simulink model "QD2_DroneStack_PID_R2023a"  (R2023a)
settings: Solver=ode1  StartTime=0.0  StopTime=inf  FixedStep=1/1000  RelTol=1e-3  EnableMultiTasking=on
InitFcn:
  | Motor_Mapping_7_Inch
model workspace (MAT data in the model file):
  target_system = 1
undefined symbols (not defined in the file): _Commander, datetime, HIL, KT, lf, log_, log_QD2_, m, Motor_Matrix, n, qc_get_step_size, s, saved_data
libraries: quarc_library x112, simulink x27, simulink_extras x3
(part 3 of 5)

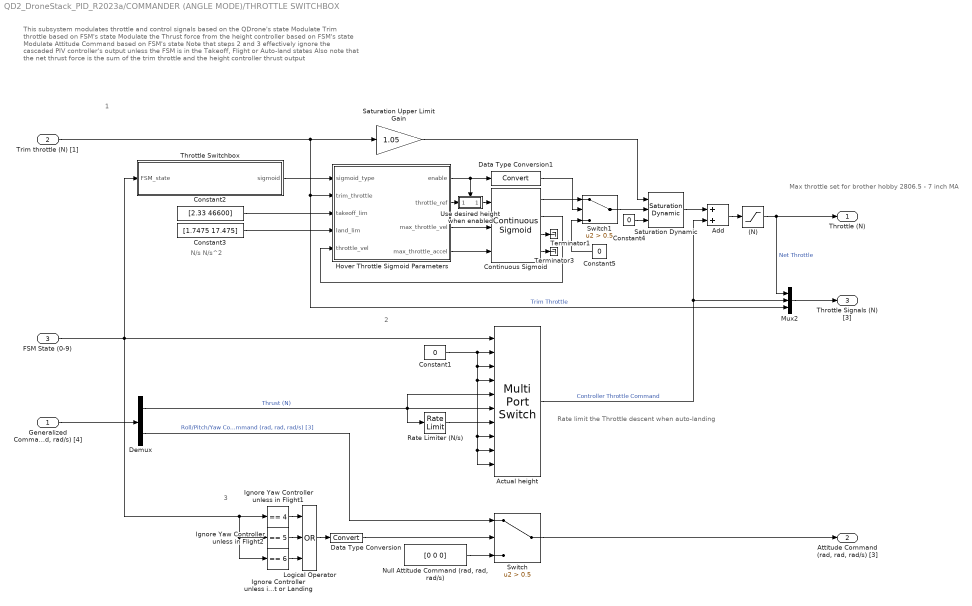
== system QD2_DroneStack_PID_R2023a/COMMANDER (ANGLE MODE)/THROTTLE SWITCHBOX  ==
  note: N/s N/s^2
  note: This subsystem modulates throttle and control signals based on the QDrone's state
      | Modulate Trim throttle based on FSM's state
      | Modulate the Thrust force from the height controller based on FSM's state
      | Modulate Attitude Command based on FSM's state
      |
      | Note that steps 2 and 3 effectively ignore the cascaded PIV controller's output unless the FSM is in the Takeoff, Flight or Auto-land states
      | Also note that the net thrust force is the sum of the trim throttle and the height controller thrust output
  note: Rate limit the Throttle descent when auto-landing
  note: 1
  note: 2
  note: 3
  note: Max throttle set for brother hobby 2806.5 - 7 inch MA
  "Generalized Command (N, rad, rad, rad/s) [4]" : Inport
  Trim throttle (N) [1] : Inport  Port=2
  FSM State (0-9) : Inport  Port=3
  (N) : Saturate  UpperLimit=58  LowerLimit=0
  Actual height : MultiPortSwitch  Inputs=9  SaturateOnIntegerOverflow=off  InputSameDT=off
  Add : Sum
  Constant1 : Constant  Value=0
  Constant2 : Constant  Value=[2.33 46600]
  Constant3 : Constant  Value=[1.7475 17.475]
  Constant4 : Constant  Value=0
  Constant5 : Constant  Value=0
  Continuous Sigmoid : quarc_library/Sources/Sigmoids/Continuous Sigmoid  params_source=External (input ports)  max_velocity=2  max_acceleration=10  initial_position=0  initial_velocity=0  hold_off=0.5  input_sample_time=-1  output_sample_time=qc_get_step_size
      settings: SourceProductName=QUARC Targets
  Data Type Conversion : DataTypeConversion  SaturateOnIntegerOverflow=off  RndMeth=Floor
  Data Type Conversion1 : DataTypeConversion  SaturateOnIntegerOverflow=off  RndMeth=Floor
  Demux : Demux  Outputs=[1 3]
  Hover Throttle Sigmoid Parameters : MATLAB Function  TreatAsAtomicUnit=on
  "Ignore Controller unless in Takeoff, Flight or Landing" : simulink/Logic and Bit Operations/Compare To Constant  relop===  const=6  OutDataTypeStr=boolean
  Ignore Yaw Controller unless in Flight1 : simulink/Logic and Bit Operations/Compare To Constant  relop===  const=4  OutDataTypeStr=boolean
  Ignore Yaw Controller unless in Flight2 : simulink/Logic and Bit Operations/Compare To Constant  relop===  const=5  OutDataTypeStr=boolean
  Logical Operator : Logic  Operator=OR  Inputs=3  AllPortsSameDT=off  OutDataTypeStr=boolean
  Mux2 : Mux  Inputs=3
  "Null Attitude Command (rad, rad, rad/s)" : Constant  Value=[0 0 0]
  Rate Limiter (N/s) : RateLimiter  RisingSlewLimit=100  FallingSlewLimit=-100  SampleTimeMode=inherited
  Saturation Dynamic : simulink/Discontinuities/Saturation Dynamic  OutMin=[]  OutMax=[]  OutDataTypeStr=Inherit: Same as second input  OutDataType=fixdt(1, 16)  OutScaling=2^-10  DoSatur=off
  Saturation Upper Limit Gain : Gain  Gain=1.05
  Switch : Switch  Criteria=u2 > Threshold  Threshold=0.5  SaturateOnIntegerOverflow=off  InputSameDT=off
  Switch1 : Switch  Criteria=u2 > Threshold  Threshold=0.5  SaturateOnIntegerOverflow=off  InputSameDT=off
  Terminator1 : Terminator
  Terminator3 : Terminator
  Throttle Switchbox : MATLAB Function  TreatAsAtomicUnit=on
  Use desired height when enabled : Subsystem  TreatAsAtomicUnit=on
  Throttle (N) : Outport  VectorParamsAs1DForOutWhenUnconnected=off
  "Attitude Command (rad, rad, rad/s) [3]" : Outport  Port=2  VectorParamsAs1DForOutWhenUnconnected=off
  Throttle Signals (N) [3] : Outport  Port=3  VectorParamsAs1DForOutWhenUnconnected=off
  wires:
  Rate Limiter (N/s)/1 -> Actual height/7
  Constant1/1 -> Actual height/2, Actual height/3, Actual height/4, Actual height/9, Actual height/10, Actual height/8
  Switch/1 -> "Attitude Command (rad, rad, rad/s) [3]"/1
  Constant5/1 -> Switch1/3
  Hover Throttle Sigmoid Parameters/2(throttle_ref) -> Use desired height when enabled/1(h_d (m) [1])
  Use desired height when enabled/1(Out1) -> Continuous Sigmoid/1
  Continuous Sigmoid/3 -> Terminator1/1
  Hover Throttle Sigmoid Parameters/1(enable) -> Use desired height when enabled/Enable, Data Type Conversion1/1
  Data Type Conversion1/1 -> Switch1/2
  Hover Throttle Sigmoid Parameters/3(max_throttle_vel) -> Continuous Sigmoid/2
  Continuous Sigmoid/4 -> Terminator3/1
  Continuous Sigmoid/1 -> Switch1/1
  Hover Throttle Sigmoid Parameters/4(max_throttle_accel) -> Continuous Sigmoid/3
  Constant2/1 -> Hover Throttle Sigmoid Parameters/3(takeoff_lim)
  Saturation Upper Limit Gain/1 -> Saturation Dynamic/1
  Throttle Switchbox/1(sigmoid) -> Hover Throttle Sigmoid Parameters/1(sigmoid_type)
  Trim throttle (N) [1]/1 -> Saturation Upper Limit Gain/1, Hover Throttle Sigmoid Parameters/2(trim_throttle), Mux2/3  "Trim Throttle"
  Switch1/1 -> Saturation Dynamic/2
  Constant3/1 -> Hover Throttle Sigmoid Parameters/4(land_lim)
  Saturation Dynamic/1 -> Add/1
  Constant4/1 -> Saturation Dynamic/3
  Continuous Sigmoid/2 -> Hover Throttle Sigmoid Parameters/5(throttle_vel)
  Demux/1 -> Actual height/5, Rate Limiter (N/s)/1, Actual height/6  "Thrust (N)"
  Logical Operator/1 -> Data Type Conversion/1
  "Ignore Controller unless in Takeoff, Flight or Landing"/1 -> Logical Operator/3
  FSM State (0-9)/1 -> Throttle Switchbox/1(FSM_state), Ignore Yaw Controller unless in Flight1/1, Ignore Yaw Controller unless in Flight2/1, "Ignore Controller unless in Takeoff, Flight or Landing"/1, Actual height/1
  Demux/2 -> Switch/1  "Roll/Pitch/Yaw Command (rad, rad, rad/s) [3]"
  Ignore Yaw Controller unless in Flight1/1 -> Logical Operator/1
  "Null Attitude Command (rad, rad, rad/s)"/1 -> Switch/3
  Data Type Conversion/1 -> Switch/2
  Ignore Yaw Controller unless in Flight2/1 -> Logical Operator/2
  Mux2/1 -> Throttle Signals (N) [3]/1
  "Generalized Command (N, rad, rad, rad/s) [4]"/1 -> Demux/1
  (N)/1 -> Throttle (N)/1, Mux2/1  "Net Throttle"
  Add/1 -> (N)/1
  Actual height/1 -> Add/2, Mux2/2  "Controller Throttle Command"

== system QD2_DroneStack_PID_R2023a/Communication/Detect Communication Loss ==
  note: Stream Loss: Check if the state is 2 and error is positive (error codes are negative). Otherwise issue a communication error.
      | OR
      | Data Loss: Check if the data is stale for a while (this is required because a connected stream may publish no new data). If stale, issue a communication error.
  State : Inport
  Error : Inport  Port=2
  Data Out : Inport  Port=3
  Clock1 : Clock
  Communication Loss : Scope  NumInputPorts=2
  Data Type Conversion4 : DataTypeConversion  SaturateOnIntegerOverflow=off  RndMeth=Floor
  Grab mission server time to detect flat lines : Selector  InputPortWidth=14  IndexOptions=Index vector (dialog)  Indices=[14]  OutputSizes=1
  Logical Operator4 : Logic  Operator=OR  AllPortsSameDT=off  OutDataTypeStr=boolean
  MATLAB Function : MATLAB Function  TreatAsAtomicUnit=on
  Terminator3 : Terminator
  Terminator5 : Terminator
  Threshold1 : quarc_library/Discontinuities/Threshold  operator=>=  param_src=Specify via dialog  threshold=0.5  duration=0.1
      settings: SourceProductName=QUARC Targets
  Threshold2 : quarc_library/Discontinuities/Threshold  operator=>=  param_src=Specify via dialog  threshold=0.5  duration=0.5
      settings: SourceProductName=QUARC Targets
  Communication Issue : Outport  VectorParamsAs1DForOutWhenUnconnected=off
  wires:
  Threshold2/1 -> Communication Loss/2, Logical Operator4/2
  Logical Operator4/1 -> Data Type Conversion4/1
  Threshold1/2 -> Terminator3/1
  MATLAB Function/2(data_loss) -> Threshold2/1
  MATLAB Function/1(stream_connection_loss) -> Threshold1/1
  Clock1/1 -> MATLAB Function/1(time)
  Threshold2/2 -> Terminator5/1
  Threshold1/1 -> Communication Loss/1, Logical Operator4/1
  Grab mission server time to detect flat lines/1 -> MATLAB Function/4(ms_time)
  Data Out/1 -> Grab mission server time to detect flat lines/1
  State/1 -> MATLAB Function/2(state)
  Error/1 -> MATLAB Function/3(error)
  Data Type Conversion4/1 -> Communication Issue/1

== system QD2_DroneStack_PID_R2023a/Communication/Triggered Subsystem ==
  Trigger : TriggerPort  VariantControl=(inherit)
  Constant : Constant
  commOK : Outport  InitialOutput=[0]
  wires:
  Constant/1 -> commOK/1

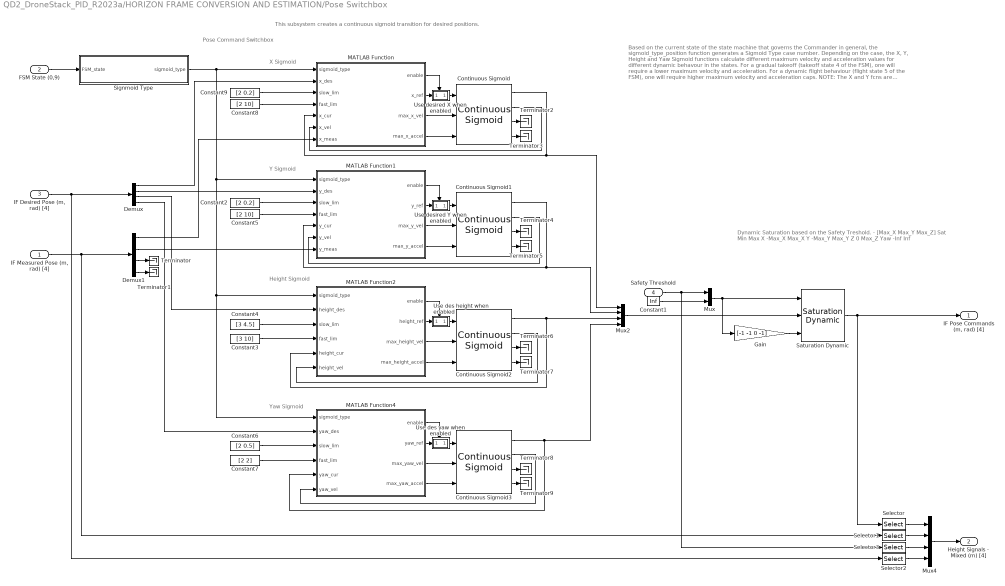
== system QD2_DroneStack_PID_R2023a/HORIZON FRAME CONVERSION AND ESTIMATION/Pose Switchbox ==
  note: Dynamic Saturation based on the Safety Treshold. - [Max_X Max_Y Max_Z]
      |
      | Sat Min Max
      | X -Max_X Max_X
      | Y -Max_Y Max_Y
      | Z 0 Max_Z
      | Yaw -Inf Inf
  note: Based on the current state of the state machine that governs the Commander in general,
      | the sigmoid_type_position function generates a Sigmoid Type case number. Depending on
      | the case, the X, Y, Height and Yaw Sigmoid functions calculate different maximum velocity
      | and acceleration values for different dynamic behavour in the states.
      |
      | For a gradual takeoff (takeoff state 4 of the FSM), one will require a lower maximum velocity
      | and acceleration. For a dynamic flight behaviour (flight state 5 of the FSM), one will require
      | higher maximum velocity and acceleration caps.
      |
      | NOTE: The X and Y fcns are logically identical due to the generally symmetric X and Y behaviour.
      | The Z and Yaw fcns are different.
  note: This subsystem creates a continuous sigmoid transition for desired positions.
  note: Height Sigmoid
  note: Pose Command Switchbox
  note: X Sigmoid
  note: Yaw Sigmoid
  note: Y Sigmoid
  "IF Measured Pose (m, rad) [4]" : Inport
  FSM State (0,9) : Inport  Port=2
  "IF Desired Pose (m, rad) [4]" : Inport  Port=3
  Safety Threshold : Inport  Port=4
  Constant1 : Constant  Value=Inf
  Constant2 : Constant  Value=[2 0.2]
  Constant3 : Constant  Value=[3 10]
  Constant4 : Constant  Value=[3 4.5]
  Constant5 : Constant  Value=[2 10]
  Constant6 : Constant  Value=[2 0.5]
  Constant7 : Constant  Value=[2 2]
  Constant8 : Constant  Value=[2 10]
  Constant9 : Constant  Value=[2 0.2]
  Continuous Sigmoid{,1..3} (4 alike) : quarc_library/Sources/Sigmoids/Continuous Sigmoid  params_source=External (input ports)  max_velocity=2  max_acceleration=10  initial_position=0  initial_velocity=0  hold_off=0.5  input_sample_time=-1  output_sample_time=qc_get_step_size
      settings: SourceProductName=QUARC Targets
  Demux : Demux
  Demux1 : Demux
  Gain : Gain  Gain=[-1 -1 0 -1]
  MATLAB Function : MATLAB Function  TreatAsAtomicUnit=on
  MATLAB Function1 : MATLAB Function  TreatAsAtomicUnit=on
  MATLAB Function2 : MATLAB Function  TreatAsAtomicUnit=on
  MATLAB Function4 : MATLAB Function  TreatAsAtomicUnit=on
  Mux : Mux  Inputs=2
  Mux2 : Mux
  Mux4 : Mux
  Saturation Dynamic : simulink/Discontinuities/Saturation Dynamic  OutMin=[]  OutMax=[]  OutDataTypeStr=Inherit: Same as second input  OutDataType=fixdt(1, 16)  OutScaling=2^-10  DoSatur=off
  Selector : Selector  InputPortWidth=4  IndexOptions=Index vector (dialog)  Indices=[3]  OutputSizes=1
  Selector1 : Selector  InputPortWidth=4  IndexOptions=Index vector (dialog)  Indices=[3]  OutputSizes=1
  Selector2 : Selector  InputPortWidth=4  IndexOptions=Index vector (dialog)  Indices=[3]  OutputSizes=1
  Selector3 : Selector  InputPortWidth=3  IndexOptions=Index vector (dialog)  Indices=[3]  OutputSizes=1
  Signmoid Type : MATLAB Function  TreatAsAtomicUnit=on
  Terminator{,1..9} (10 alike) : Terminator
  Use des height when enabled : Subsystem  TreatAsAtomicUnit=on
  Use des yaw when enabled : Subsystem  TreatAsAtomicUnit=on
  Use desired X when enabled : Subsystem  TreatAsAtomicUnit=on
  Use desired Y when enabled : Subsystem  TreatAsAtomicUnit=on
  "IF Pose Commands (m, rad) [4]" : Outport  VectorParamsAs1DForOutWhenUnconnected=off
  Height Signals - Mixed (m) [4] : Outport  Port=2  VectorParamsAs1DForOutWhenUnconnected=off
  wires:
  Constant4/1 -> MATLAB Function2/3(slow_lim)
  Constant3/1 -> MATLAB Function2/4(fast_lim)
  Selector/1 -> Mux4/1
  Selector1/1 -> Mux4/2
  Selector2/1 -> Mux4/4
  Selector3/1 -> Mux4/3
  Safety Threshold/1 -> Mux/1, Selector3/1
  Mux/1 -> Saturation Dynamic/1, Gain/1
  Constant1/1 -> Mux/2
  Saturation Dynamic/1 -> "IF Pose Commands (m, rad) [4]"/1, Selector/1
  Mux2/1 -> Saturation Dynamic/2
  Mux4/1 -> Height Signals - Mixed (m) [4]/1
  Gain/1 -> Saturation Dynamic/3
  Demux/2 -> MATLAB Function1/2(y_des)
  Use desired Y when enabled/1(Out1) -> Continuous Sigmoid1/1
  Use desired X when enabled/1(Out1) -> Continuous Sigmoid/1
  MATLAB Function2/3(max_height_vel) -> Continuous Sigmoid2/2
  Continuous Sigmoid3/3 -> Terminator8/1
  Demux1/4 -> Terminator1/1
  MATLAB Function4/1(enable) -> Use des yaw when enabled/Enable
  Use des yaw when enabled/1(Out1) -> Continuous Sigmoid3/1
  Continuous Sigmoid1/2 -> MATLAB Function1/6(y_vel)
  Constant2/1 -> MATLAB Function1/3(slow_lim)
  Constant6/1 -> MATLAB Function4/3(slow_lim)
  Demux1/1 -> MATLAB Function/7(x_meas)
  MATLAB Function1/2(y_ref) -> Use desired Y when enabled/1(h_d (m) [1])
  Demux/3 -> MATLAB Function2/2(height_des)
  Constant7/1 -> MATLAB Function4/4(fast_lim)
  Continuous Sigmoid1/4 -> Terminator5/1
  MATLAB Function1/1(enable) -> Use desired Y when enabled/Enable
  Continuous Sigmoid2/4 -> Terminator7/1
  Demux1/3 -> Terminator/1
  Signmoid Type/1(sigmoid_type) -> MATLAB Function/1(sigmoid_type), MATLAB Function1/1(sigmoid_type), MATLAB Function2/1(sigmoid_type), MATLAB Function4/1(sigmoid_type)
  MATLAB Function/3(max_x_vel) -> Continuous Sigmoid/2
  MATLAB Function2/1(enable) -> Use des height when enabled/Enable
  Constant9/1 -> MATLAB Function/3(slow_lim)
  Continuous Sigmoid2/2 -> MATLAB Function2/6(height_vel)
  Continuous Sigmoid1/1 -> MATLAB Function1/5(y_cur), Mux2/2
  MATLAB Function4/4(max_yaw_accel) -> Continuous Sigmoid3/3
  Demux/1 -> MATLAB Function/2(x_des)
  MATLAB Function1/3(max_y_vel) -> Continuous Sigmoid1/2
  Continuous Sigmoid3/2 -> MATLAB Function4/6(yaw_vel)
  MATLAB Function2/2(height_ref) -> Use des height when enabled/1(h_d (m) [1])
  MATLAB Function/4(max_x_accel) -> Continuous Sigmoid/3
  Use des height when enabled/1(Out1) -> Continuous Sigmoid2/1
  Continuous Sigmoid2/3 -> Terminator6/1
  Demux/4 -> MATLAB Function4/2(yaw_des)
  MATLAB Function1/4(max_y_accel) -> Continuous Sigmoid1/3
  MATLAB Function/1(enable) -> Use desired X when enabled/Enable
  Continuous Sigmoid3/4 -> Terminator9/1
  MATLAB Function4/2(yaw_ref) -> Use des yaw when enabled/1(h_d (m) [1])
  FSM State (0,9)/1 -> Signmoid Type/1(FSM_state)
  MATLAB Function2/4(max_height_accel) -> Continuous Sigmoid2/3
  Continuous Sigmoid/4 -> Terminator3/1
  Continuous Sigmoid/3 -> Terminator2/1
  Continuous Sigmoid/1 -> MATLAB Function/5(x_cur), Mux2/1
  Continuous Sigmoid/2 -> MATLAB Function/6(x_vel)
  MATLAB Function/2(x_ref) -> Use desired X when enabled/1(h_d (m) [1])
  Continuous Sigmoid3/1 -> MATLAB Function4/5(yaw_cur), Mux2/4
  MATLAB Function4/3(max_yaw_vel) -> Continuous Sigmoid3/2
  Continuous Sigmoid2/1 -> MATLAB Function2/5(height_cur), Mux2/3
  Demux1/2 -> MATLAB Function1/7(y_meas)
  Continuous Sigmoid1/3 -> Terminator4/1
  "IF Measured Pose (m, rad) [4]"/1 -> Demux1/1, Selector1/1
  "IF Desired Pose (m, rad) [4]"/1 -> Demux/1, Selector2/1
  Constant5/1 -> MATLAB Function1/4(fast_lim)
  Constant8/1 -> MATLAB Function/4(fast_lim)

== system QD2_DroneStack_PID_R2023a/QDrone 2 DAQ/Attitude Estimate from IMU Data ==
  IMU Data [12] : Inport
  For Each Subsystem - Iterate over IMU0 and IMU1 : Subsystem  TreatAsAtomicUnit=on
  Reshape into 2 columns for IMU0 and IMU1 : Reshape  OutputDimensionality=Customize  OutputDimensions=[6,2]
  Select Data for IMU0 : Selector  NumberOfDimensions=2  InputPortWidth=3  IndexOptions=Index vector (dialog),Index vector (dialog)  Indices=[1:9],[1]  OutputSizes=1,1
  Select Data for IMU1 : Selector  NumberOfDimensions=2  InputPortWidth=3  IndexOptions=Index vector (dialog),Index vector (dialog)  Indices=[1:9],[2]  OutputSizes=1,1
  "BF Estimated Attitude for IMU0 (rad, rad/s, rad/2^2) [9]" : Outport
  "BF Estimated Attitude for IMU1 (rad, rad/s, rad/2^2) [9]" : Outport  Port=2
  wires:
  Select Data for IMU1/1 -> "BF Estimated Attitude for IMU1 (rad, rad/s, rad/2^2) [9]"/1
  Select Data for IMU0/1 -> "BF Estimated Attitude for IMU0 (rad, rad/s, rad/2^2) [9]"/1
  For Each Subsystem - Iterate over IMU0 and IMU1/1("BF Estimated Attitude (rad, rad/s, rad/2^2) [9xn]") -> Select Data for IMU0/1, Select Data for IMU1/1
  Reshape into 2 columns for IMU0 and IMU1/1 -> For Each Subsystem - Iterate over IMU0 and IMU1/1(IMU Data [6xn])
  IMU Data [12]/1 -> Reshape into 2 columns for IMU0 and IMU1/1

== system QD2_DroneStack_PID_R2023a/QDrone 2 DAQ/Choose Motor Telemetry ==
  enable telemetry : Inport
  Bias1 : Bias  Bias=0:3  SaturateOnIntegerOverflow=off
  Constant1 : Constant  Value="[0 0 0 0; 1 0 0 0; 0 0 0 0; 0 1 0 0; 0 0 0 0; 0 0 1 0; 0 0 0 0;  0 0 0 1]"
  Constant2 : Constant  Value=8
  Gain : Gain  Gain=.7
  MATLAB Function : MATLAB Function  TreatAsAtomicUnit=on
  Selector : Selector  NumberOfDimensions=2  IndexMode=Zero-based  InputPortWidth=3  IndexOptions=Index vector (port),Select all  Indices=[1 3],1  OutputSizes=1,1
  Telemetry : Scope
  Zero-Order Hold1 : ZeroOrderHold  SampleTime=-1
  Motor telemetry select : Outport
  Motor telemetry index : Outport  Port=2
  wires:
  Constant2/1 -> MATLAB Function/2(n)
  Constant1/1 -> Selector/1
  Selector/1 -> Gain/1, Motor telemetry select/1
  enable telemetry/1 -> MATLAB Function/1(enable)
  Zero-Order Hold1/1 -> Motor telemetry index/1, Selector/2
  MATLAB Function/1(idx) -> Zero-Order Hold1/1
  Bias1/1 -> Telemetry/1
  Gain/1 -> Bias1/1

== system QD2_DroneStack_PID_R2023a/QDrone 2 DAQ/Construct ESC Speed ==
  ESC Data In [4] : Inport
  ESC Channel Select : Inport  Port=2
  For Each Subsystem - Construct ESC Signal : Subsystem  TreatAsAtomicUnit=on
  Memory : Memory  InitialCondition=zeros(1,4)
  ESC Data Out [4] : Outport
  wires:
  ESC Channel Select/1 -> For Each Subsystem - Construct ESC Signal/2(ESC Channel)
  ESC Data In [4]/1 -> For Each Subsystem - Construct ESC Signal/1(ESC Data In [4])
  Memory/1 -> For Each Subsystem - Construct ESC Signal/3(ESC Previous Data [4])
  For Each Subsystem - Construct ESC Signal/1(ESC Data Out [4]) -> Memory/1, ESC Data Out [4]/1

== system QD2_DroneStack_PID_R2023a/QDrone 2 DAQ/Construct ESC Temperature ==
  ESC Data In [4] : Inport
  ESC Channel Select : Inport  Port=2
  For Each Subsystem - Construct ESC Signal : Subsystem  TreatAsAtomicUnit=on
  Memory : Memory  InitialCondition=zeros(1,4)
  ESC Data Out [4] : Outport
  wires:
  ESC Channel Select/1 -> For Each Subsystem - Construct ESC Signal/2(ESC Channel)
  ESC Data In [4]/1 -> For Each Subsystem - Construct ESC Signal/1(ESC Data In [4])
  Memory/1 -> For Each Subsystem - Construct ESC Signal/3(ESC Previous Data [4])
  For Each Subsystem - Construct ESC Signal/1(ESC Data Out [4]) -> Memory/1, ESC Data Out [4]/1

== system QD2_DroneStack_PID_R2023a/QDrone 2 DAQ/Construct ESC Voltage ==
  ESC Data In [4] : Inport
  ESC Channel Select : Inport  Port=2
  For Each Subsystem - Construct ESC Signal : Subsystem  TreatAsAtomicUnit=on
  Memory : Memory  InitialCondition=zeros(1,4)
  ESC Data Out [4] : Outport
  wires:
  For Each Subsystem - Construct ESC Signal/1(ESC Data Out [4]) -> ESC Data Out [4]/1, Memory/1
  Memory/1 -> For Each Subsystem - Construct ESC Signal/3(ESC Previous Data [4])
  ESC Data In [4]/1 -> For Each Subsystem - Construct ESC Signal/1(ESC Data In [4])
  ESC Channel Select/1 -> For Each Subsystem - Construct ESC Signal/2(ESC Channel)

== system QD2_DroneStack_PID_R2023a/QDrone 2 DAQ/Detect ESC Problems ==
  ESC Telemetry Enabled : Inport
  ESC Channel Request [4] : Inport  Port=2
  ESC Channel Reported [4] : Inport  Port=3
  AND : Logic  IconShape=distinctive  AllPortsSameDT=off  OutDataTypeStr=boolean
  Compare To Constant : simulink/Logic and Bit Operations/Compare To Constant  relop=>=  const=20  OutDataTypeStr=boolean
  Constant : Constant  Value=200
  Delay{,1..3} (4 alike) : Delay
  Demux{,1..2,8} (4 alike) : Demux
  ESC Channel Mismatrch : Scope  NumInputPorts=4
  ESC Channel Mismatrch Count : Scope  NumInputPorts=4
  ESC Channel Selection Index : Scope  NumInputPorts=4
  For Each Subsystem : Subsystem  TreatAsAtomicUnit=on
  MATLAB Function : MATLAB Function  TreatAsAtomicUnit=on
  Mux : Mux
  Mux{1..4} (4 alike) : Mux  Inputs=2
  ESC Comm Problem [4] : Outport
  wires:
  Mux1/1 -> ESC Channel Selection Index/4
  Mux2/1 -> ESC Channel Selection Index/3
  Mux3/1 -> ESC Channel Selection Index/2
  Mux4/1 -> ESC Channel Selection Index/1
  Demux2/4 -> Mux4/2
  Demux2/3 -> Mux3/2
  Demux2/2 -> Mux2/2
  Demux2/1 -> Mux1/2
  ESC Telemetry Enabled/1 -> AND/2
  Compare To Constant/1 -> ESC Comm Problem [4]/1
  MATLAB Function/1(n) -> Demux1/1, Compare To Constant/1
  Demux1/2 -> ESC Channel Mismatrch Count/3
  Demux1/1 -> ESC Channel Mismatrch Count/4
  Demux1/3 -> ESC Channel Mismatrch Count/2
  Demux1/4 -> ESC Channel Mismatrch Count/1
  Constant/1 -> MATLAB Function/2(buffer_size)
  Demux8/4 -> ESC Channel Mismatrch/1
  Demux8/3 -> ESC Channel Mismatrch/2
  Demux8/1 -> ESC Channel Mismatrch/4
  Demux8/2 -> ESC Channel Mismatrch/3
  AND/1 -> Demux8/1, MATLAB Function/1(u)
  For Each Subsystem/1(mismatched [4]) -> AND/1
  Mux/1 -> For Each Subsystem/1(Channel Requested [4])
  Delay/1 -> Mux/4, Mux4/1
  Delay1/1 -> Mux/3, Mux3/1
  Delay3/1 -> Mux1/1, Mux/1
  Delay2/1 -> Mux/2, Mux2/1
  ESC Channel Request [4]/1 -> Demux/1
  Demux/4 -> Delay/1
  Demux/3 -> Delay1/1
  Demux/2 -> Delay2/1
  Demux/1 -> Delay3/1
  ESC Channel Reported [4]/1 -> For Each Subsystem/2(Channel Reported [4]), Demux2/1

== system QD2_DroneStack_PID_R2023a/QDrone 2 DAQ/Enabled Subsystem - Write ESC Commands ==
  DShot Raw [4] : Inport
  Enable : EnablePort
  HIL Write PWM : quarc_library/Data Acquisition/Generic/Immediate I//O/HIL Write PWM  object_name=HIL-1  channels=[0:3]  sample_time=-1  active=off  vector_input=on
      settings: AttributesFormatString=(%<object_name>)  SourceProductName=QUARC Targets
  wires:
  DShot Raw [4]/1 -> HIL Write PWM/1

== system QD2_DroneStack_PID_R2023a/QDrone 2 DAQ/Generate LED Pattern ==
  ESC States : Inport
  Blue Blue : Constant  Value=[0 0 1 0 0 1]
  Green Green : Constant  Value=[0 1 0 0 1 0]
  LED OFF : Constant  Value=[ 0 0 0 0 0 0]
  Multiport Switch : MultiPortSwitch  DataPortOrder=Specify indices  DataPortIndices={0,1,2,3,4,5,77,88,99}  DataPortForDefault=Additional data port  DiagnosticForDefault=Warning  SaturateOnIntegerOverflow=off  InputSameDT=off
  Red Blue : Constant  Value="[ 1 0 0 0 0 1   ]"
  Red Red : Constant  Value=[ 1 0 0 1 0 0]
  Red Yellow : Constant  Value="[ 1 0 0 1 1 0  ]"
  Yellow Blue : Constant  Value="[ 1 1 0 0 0 1  ]"
  Yellow Green : Constant  Value="[ 1 1 0 0 1 0  ]"
  Yellow Red : Constant  Value="[ 1 1 0 1 0 0  ]"
  Yellow Yellow : Constant  Value="[ 1 1 0 1 1 0  ]"
  LED Command : Outport
  wires:
  Red Yellow/1 -> Multiport Switch/6
  Yellow Red/1 -> Multiport Switch/5
  Yellow Green/1 -> Multiport Switch/3
  Green Green/1 -> Multiport Switch/7
  LED OFF/1 -> Multiport Switch/11
  Yellow Blue/1 -> Multiport Switch/8
  Red Blue/1 -> Multiport Switch/9
  Yellow Yellow/1 -> Multiport Switch/2
  Red Red/1 -> Multiport Switch/10
  Blue Blue/1 -> Multiport Switch/4
  ESC States/1 -> Multiport Switch/1
  Multiport Switch/1 -> LED Command/1

== system QD2_DroneStack_PID_R2023a/QDrone 2 DAQ/Monitor Battery Level ==
  note: Monitor Battery Level.
      | Flag Low Battery Error if
      | Battery level dips below
      | threshold for specified
      | threshold time period.
  Battery (V) : Inport
  AND : Logic  IconShape=distinctive  AllPortsSameDT=off  OutDataTypeStr=boolean
  Battery Low Time Threshold (s) : Constant  Value=0.3
  Constant : Constant  Value=0.5
  Data Type Conversion : DataTypeConversion  SaturateOnIntegerOverflow=off  RndMeth=Floor
  Data Type Conversion1 : DataTypeConversion  SaturateOnIntegerOverflow=off  RndMeth=Floor
  Greater than minimum expected voltage (Valid Battery Reading) : simulink/Logic and Bit Operations/Compare To Constant  relop=>  const=0.5  OutDataTypeStr=boolean
  Less than minimum threshold voltage (Battery level too low) : simulink/Logic and Bit Operations/Compare To Constant  relop=<=  const=14  OutDataTypeStr=boolean
  Terminator : Terminator
  Threshold : quarc_library/Discontinuities/Threshold  operator=>=  param_src=External input port  threshold=0  duration=0
      settings: SourceProductName=QUARC Targets
  Triggered Subsystem - Latching Flag : Subsystem  TreatAsAtomicUnit=on
  Low Battery : Outport
  wires:
  Data Type Conversion1/1 -> Low Battery/1
  Triggered Subsystem - Latching Flag/1(Out1) -> Data Type Conversion1/1
  Threshold/1 -> Triggered Subsystem - Latching Flag/Trigger
  Threshold/2 -> Terminator/1
  Data Type Conversion/1 -> Threshold/1
  Battery Low Time Threshold (s)/1 -> Threshold/3
  Constant/1 -> Threshold/2
  AND/1 -> Data Type Conversion/1
  Greater than minimum expected voltage (Valid Battery Reading)/1 -> AND/1
  Less than minimum threshold voltage (Battery level too low)/1 -> AND/2
  Battery (V)/1 -> Greater than minimum expected voltage (Valid Battery Reading)/1, Less than minimum threshold voltage (Battery level too low)/1

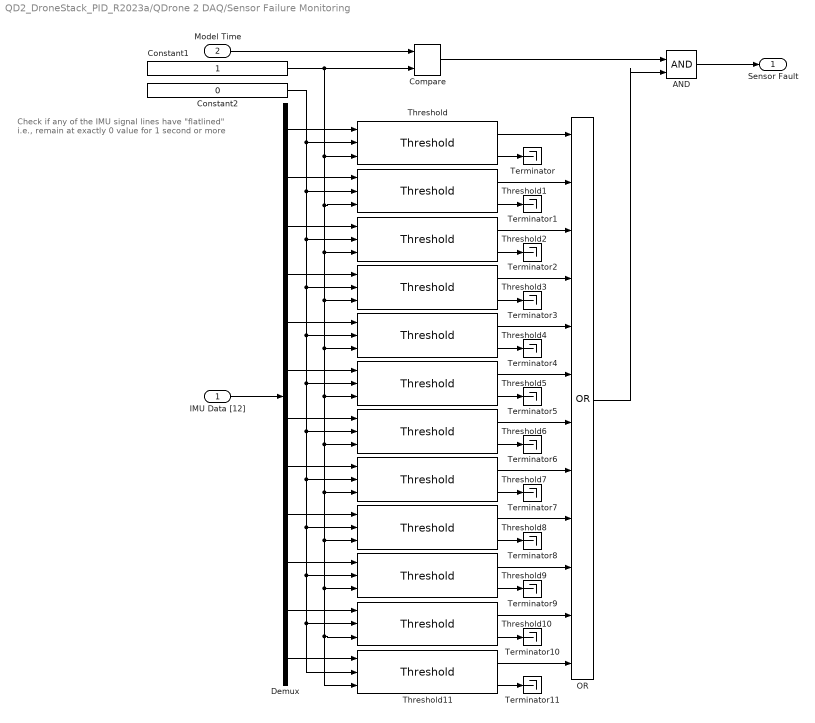
== system QD2_DroneStack_PID_R2023a/QDrone 2 DAQ/Sensor Failure Monitoring ==
  note: Check if any of the IMU signal lines have "flatlined"
      | i.e., remain at exactly 0 value for 1 second or more
  IMU Data [12] : Inport
  Model Time : Inport  Port=2
  AND : Logic  IconShape=distinctive  AllPortsSameDT=off  OutDataTypeStr=boolean
  Compare : quarc_library/Logic Operations/Compare  operator=>=  output_data_type=boolean
      settings: SourceProductName=QUARC Targets
  Constant1 : Constant
  Constant2 : Constant  Value=0
  Demux : Demux  Outputs=12
  OR : Logic  Operator=OR  Inputs=12  AllPortsSameDT=off  OutDataTypeStr=boolean
  Terminator{,1..11} (12 alike) : Terminator
  Threshold{,1..11} (12 alike) : quarc_library/Discontinuities/Threshold  operator===  param_src=External input port  threshold=0  duration=1
      settings: SourceProductName=QUARC Targets
  Sensor Fault : Outport
  wires:
  AND/1 -> Sensor Fault/1
  OR/1 -> AND/2
  Compare/1 -> AND/1
  Threshold11/2 -> Terminator11/1
  Threshold10/2 -> Terminator10/1
  Threshold9/2 -> Terminator9/1
  Threshold8/2 -> Terminator8/1
  Threshold7/2 -> Terminator7/1
  Threshold6/2 -> Terminator6/1
  Threshold5/2 -> Terminator5/1
  Threshold4/2 -> Terminator4/1
  Threshold3/2 -> Terminator3/1
  Threshold2/2 -> Terminator2/1
  Threshold1/2 -> Terminator1/1
  Threshold/2 -> Terminator/1
  Threshold11/1 -> OR/12
  Threshold10/1 -> OR/11
  Threshold9/1 -> OR/10
  Threshold8/1 -> OR/9
  Threshold7/1 -> OR/8
  Threshold6/1 -> OR/7
  Threshold5/1 -> OR/6
  Threshold4/1 -> OR/5
  Threshold3/1 -> OR/4
  Threshold2/1 -> OR/3
  Threshold1/1 -> OR/2
  Threshold/1 -> OR/1
  Demux/12 -> Threshold11/1
  Demux/11 -> Threshold10/1
  Demux/10 -> Threshold9/1
  Demux/9 -> Threshold8/1
  Demux/8 -> Threshold7/1
  Demux/7 -> Threshold6/1
  Demux/6 -> Threshold5/1
  Demux/5 -> Threshold4/1
  Demux/4 -> Threshold3/1
  Demux/3 -> Threshold2/1
  IMU Data [12]/1 -> Demux/1
  Constant2/1 -> Threshold/2, Threshold11/2, Threshold10/2, Threshold9/2, Threshold8/2, Threshold7/2, Threshold6/2, Threshold5/2, Threshold4/2, Threshold3/2, Threshold2/2, Threshold1/2
  Demux/2 -> Threshold1/1
  Demux/1 -> Threshold/1
  Constant1/1 -> Compare/2, Threshold/3, Threshold4/3, Threshold11/3, Threshold10/3, Threshold9/3, Threshold8/3, Threshold7/3, Threshold6/3, Threshold5/3, Threshold3/3, Threshold2/3, Threshold1/3
  Model Time/1 -> Compare/1

== system QD2_DroneStack_PID_R2023a/QDrone 2 DAQ/Timing Monitors ==
  note: ToF Range Rate (25 Hz)
  note: Optical Flow Rate (100 Hz)
  note: Base Model Rate (1kHz)
  Computation Time : quarc_library/Sources/Time/Computation Time  sample_time=qc_get_step_size  use_model=on  use_cpu_time=off
  Computation Time1 : quarc_library/Sources/Time/Computation Time  sample_time=0.01  use_model=on  use_cpu_time=off
  Computation Time2 : quarc_library/Sources/Time/Computation Time  sample_time=0.04  use_model=on  use_cpu_time=off
  Mux : Mux  Inputs=2
  Mux1 : Mux  Inputs=2
  Mux2 : Mux  Inputs=2
  Mux3 : Mux  Inputs=3
  Rate Transition{,1..3} (4 alike) : RateTransition
  Sample Time : quarc_library/Sources/Time/Sample Time  Priority=-99  sample_time=qc_get_step_size
  Sample Time1 : quarc_library/Sources/Time/Sample Time  Priority=-99  sample_time=0.01
  Sample Time2 : quarc_library/Sources/Time/Sample Time  Priority=-99  sample_time=0.04
  Timing Check : Scope  NumInputPorts=3
  Timings : Outport
  wires:
  Rate Transition3/1 -> Mux2/2
  Rate Transition2/1 -> Mux2/1
  Rate Transition1/1 -> Mux1/2
  Rate Transition/1 -> Mux1/1
  Mux3/1 -> Timings/1
  Mux2/1 -> Mux3/3, Timing Check/3
  Mux/1 -> Mux3/1, Timing Check/1
  Mux1/1 -> Timing Check/2, Mux3/2
  Sample Time2/1 -> Rate Transition3/1
  Computation Time2/1 -> Rate Transition2/1
  Computation Time1/1 -> Rate Transition/1
  Sample Time1/1 -> Rate Transition1/1
  Sample Time/1 -> Mux/2
  Computation Time/1 -> Mux/1

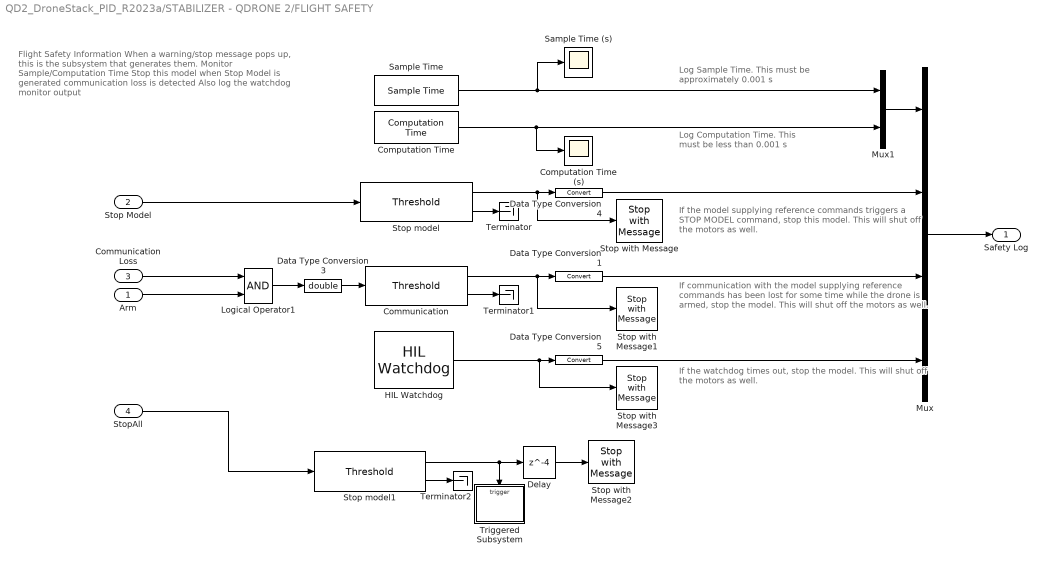
== system QD2_DroneStack_PID_R2023a/STABILIZER - QDRONE 2/FLIGHT SAFETY ==
  note: If the watchdog times out, stop the model. This will shut off the motors as well.
  note: If communication with the model supplying reference commands has been lost for some time while the drone is armed, stop the model. This will shut off the motors as well.
  note: If the model supplying reference commands triggers a STOP MODEL command, stop this model. This will shut off the motors as well.
  note: Log Computation Time. This must be less than 0.001 s
  note: Log Sample Time. This must be approximately 0.001 s
  note: Flight Safety Information
      |
      | When a warning/stop message pops up, this is the subsystem
      | that generates them.
      |
      | Monitor Sample/Computation Time
      | Stop this model
      | when Stop Model is generated
      | communication loss is detected
      | Also log the watchdog monitor output
  Arm : Inport
  Stop Model : Inport  Port=2
  Communication Loss : Inport  Port=3
  StopAll : Inport  Port=4
  Communication : quarc_library/Discontinuities/Threshold  operator=>=  param_src=Specify via dialog  threshold=0.5  duration=1
      settings: SourceProductName=QUARC Targets
  Computation Time : quarc_library/Sources/Time/Computation Time  sample_time=qc_get_step_size  use_model=on  use_cpu_time=off
  Computation Time (s) : Scope
  Data Type Conversion1 : DataTypeConversion  SaturateOnIntegerOverflow=off  RndMeth=Floor
  Data Type Conversion3 : DataTypeConversion  OutDataTypeStr=double  SaturateOnIntegerOverflow=off  RndMeth=Floor
  Data Type Conversion4 : DataTypeConversion  SaturateOnIntegerOverflow=off  RndMeth=Floor
  Data Type Conversion5 : DataTypeConversion  SaturateOnIntegerOverflow=off  RndMeth=Floor
  Delay : Delay  DelayLength=4
  HIL Watchdog : quarc_library/Data Acquisition/Generic/Watchdog/HIL Watchdog  object_name=HIL-1  timeout=0.1  sample_time=qc_get_step_size  active=off
      settings: AttributesFormatString=(%<object_name>)  SourceProductName=QUARC Targets
  Logical Operator1 : Logic  AllPortsSameDT=off  OutDataTypeStr=boolean
  Mux : Mux
  Mux1 : Mux  Inputs=2
  Sample Time : quarc_library/Sources/Time/Sample Time  Priority=-99  sample_time=qc_get_step_size
  Sample Time (s) : Scope
  Stop model : quarc_library/Discontinuities/Threshold  operator=>=  param_src=Specify via dialog  threshold=0.5  duration=0.2
      settings: SourceProductName=QUARC Targets
  Stop model1 : quarc_library/Discontinuities/Threshold  operator=>=  param_src=Specify via dialog  threshold=0.5  duration=1
      settings: SourceProductName=QUARC Targets
  Stop with Message : quarc_library/Sinks/Error Handling/Stop with Message  message_type=Fixed error message  message_icon=Information  message=QDrone Stabilizer: Commander Terminated
  Stop with Message1 : quarc_library/Sinks/Error Handling/Stop with Message  message_type=Fixed error message  message_icon=Warning  message=QDrone Stabilizer: Communication with Commander lost
  Stop with Message2 : quarc_library/Sinks/Error Handling/Stop with Message  message_type=Fixed error message  message_icon=Information  message=QDrone Stabilizer stopped from Mission Server
  Stop with Message3 : quarc_library/Sinks/Error Handling/Stop with Message  message_type=Fixed error message  message_icon=Information  message=QDrone Stabilizer: HIL Watchdog timer expired
  Terminator : Terminator
  Terminator1 : Terminator
  Terminator2 : Terminator
  Triggered Subsystem : Subsystem  TreatAsAtomicUnit=on
  Safety Log : Outport  VectorParamsAs1DForOutWhenUnconnected=off
  wires:
  Data Type Conversion5/1 -> Mux/4
  Mux1/1 -> Mux/1
  Communication Loss/1 -> Logical Operator1/1
  Data Type Conversion3/1 -> Communication/1
  Communication/1 -> Stop with Message1/1, Data Type Conversion1/1
  Arm/1 -> Logical Operator1/2
  Data Type Conversion1/1 -> Mux/3
  Logical Operator1/1 -> Data Type Conversion3/1
  Communication/2 -> Terminator1/1
  Stop Model/1 -> Stop model/1
  Stop model/1 -> Stop with Message/1, Data Type Conversion4/1
  Stop model/2 -> Terminator/1
  HIL Watchdog/1 -> Data Type Conversion5/1, Stop with Message3/1
  Data Type Conversion4/1 -> Mux/2
  Sample Time/1 -> Mux1/1, Sample Time (s)/1
  Computation Time/1 -> Mux1/2, Computation Time (s)/1
  Mux/1 -> Safety Log/1
  StopAll/1 -> Stop model1/1
  Stop model1/1 -> Delay/1, Triggered Subsystem/Trigger
  Stop model1/2 -> Terminator2/1
  Delay/1 -> Stop with Message2/1

== system QD2_DroneStack_PID_R2023a/COMMANDER (ANGLE MODE)/STATE MACHINE SIGNALS/Generate Extra Messages for Console ==
  time (s) : Inport
  Signal Triggers : Inport  Port=2
  Boolean Edge-Based Triggered Print : Subsystem  TreatAsAtomicUnit=on
  Matrix Concatenate : Concatenate  NumInputs=3  Mode=Multidimensional array  ConcatenateDimension=2
  String Constant12 : quarc_library/Strings/String Constant  string_value=DRONE DISARMED  evaluate_string=off  string_type=text  max_length=80  sample_time=inf  variable_size=off
      settings: AttributesFormatString="\"DRONE DISARMED\""  SourceProductName=QUARC Targets
  String Constant13 : quarc_library/Strings/String Constant  string_value=DRONE LANDING  evaluate_string=off  string_type=text  max_length=80  sample_time=inf  variable_size=off
      settings: AttributesFormatString="\"DRONE LANDING\""  SourceProductName=QUARC Targets
  String Constant16 : quarc_library/Strings/String Constant  string_value=INITIALIZATION FINISHED  evaluate_string=off  string_type=text  max_length=80  sample_time=inf  variable_size=off
      settings: AttributesFormatString="\"INITIALIZATION FINISHED\""  SourceProductName=QUARC Targets
  Terminator : Terminator
  wires:
  Matrix Concatenate/1 -> Boolean Edge-Based Triggered Print/2(Message)
  time (s)/1 -> Boolean Edge-Based Triggered Print/3(time (s))
  Signal Triggers/1 -> Boolean Edge-Based Triggered Print/1(Signal Enable)
  String Constant16/1 -> Matrix Concatenate/1
  String Constant12/1 -> Matrix Concatenate/2
  String Constant13/1 -> Matrix Concatenate/3
  Boolean Edge-Based Triggered Print/1(Out1) -> Terminator/1

== system QD2_DroneStack_PID_R2023a/COMMANDER (ANGLE MODE)/STATE MACHINE SIGNALS/Generate State Messages for Console ==
  time (s) : Inport
  DroneState [1-9] : Inport  Port=2
  Detect Change : simulink/Logic and Bit Operations/Detect Change  vinit=0  OutDataTypeStr=boolean
  Multiport Switch : MultiPortSwitch  Inputs=9  SaturateOnIntegerOverflow=off  InputSameDT=off
  String Constant1 : quarc_library/Strings/String Constant  string_value=DRONE ARMED  evaluate_string=off  string_type=text  max_length=80  sample_time=inf  variable_size=off
      settings: AttributesFormatString="\"DRONE ARMED\""  SourceProductName=QUARC Targets
  String Constant2 : quarc_library/Strings/String Constant  string_value=DRONE TAKEOFF THROTTLE  evaluate_string=off  string_type=text  max_length=80  sample_time=inf  variable_size=off
      settings: AttributesFormatString="\"DRONE TAKEOFF THROTTLE\""  SourceProductName=QUARC Targets
  String Constant3 : quarc_library/Strings/String Constant  string_value=DRONE TAKEOFF HEIGHT STATE  evaluate_string=off  string_type=text  max_length=80  sample_time=inf  variable_size=off
      settings: AttributesFormatString="\"DRONE TAKEOFF HEIGHT STATE\""  SourceProductName=QUARC Targets
  String Constant4 : quarc_library/Strings/String Constant  string_value=ERROR - DRONE EMERGENCY STOP  evaluate_string=off  string_type=text  max_length=80  sample_time=inf  variable_size=off
      settings: AttributesFormatString="\"ERROR - DRONE EMERGENCY STOP\""  SourceProductName=QUARC Targets
  String Constant5 : quarc_library/Strings/String Constant  string_value=DRONE IDLE - WAITING TO BE ARMED  evaluate_string=off  string_type=text  max_length=80  sample_time=inf  variable_size=off
      settings: AttributesFormatString="\"DRONE IDLE - WAITING TO BE ARMED\""  SourceProductName=QUARC Targets
  String Constant6 : quarc_library/Strings/String Constant  string_value=DRONE IS IN FLIGHT STATE  evaluate_string=off  string_type=text  max_length=80  sample_time=inf  variable_size=off
      settings: AttributesFormatString="\"DRONE IS IN FLIGHT STATE\""  SourceProductName=QUARC Targets
  String Constant7 : quarc_library/Strings/String Constant  string_value=EMERGENCY STOP WAS PRESSED ON JOYSTICK  evaluate_string=off  string_type=text  max_length=80  sample_time=inf  variable_size=off
      settings: AttributesFormatString="\"EMERGENCY STOP WAS PRESSED ON JOYSTICK\""  SourceProductName=QUARC Targets
  String Constant8 : quarc_library/Strings/String Constant  string_value=FLIGHT FINISHED DRONE IS DISABLED  evaluate_string=off  string_type=text  max_length=80  sample_time=inf  variable_size=off
      settings: AttributesFormatString="\"FLIGHT FINISHED DRONE IS DISABLED\""  SourceProductName=QUARC Targets
  String Constant9 : quarc_library/Strings/String Constant  string_value=DRONE IS AUTO LANDING  evaluate_string=off  string_type=text  max_length=80  sample_time=inf  variable_size=off
      settings: AttributesFormatString="\"DRONE IS AUTO LANDING\""  SourceProductName=QUARC Targets
  Triggered Subsystem : Subsystem  TreatAsAtomicUnit=on
  wires:
  DroneState [1-9]/1 -> Multiport Switch/1, Triggered Subsystem/1(Value), Detect Change/1
  Multiport Switch/1 -> Triggered Subsystem/3(Message)
  time (s)/1 -> Triggered Subsystem/2(Time (s))
  String Constant1/1 -> Multiport Switch/3
  String Constant2/1 -> Multiport Switch/4
  String Constant3/1 -> Multiport Switch/5
  String Constant6/1 -> Multiport Switch/6
  String Constant9/1 -> Multiport Switch/7
  String Constant4/1 -> Multiport Switch/8
  String Constant7/1 -> Multiport Switch/9
  String Constant8/1 -> Multiport Switch/10
  String Constant5/1 -> Multiport Switch/2
  Detect Change/1 -> Triggered Subsystem/Trigger

== system QD2_DroneStack_PID_R2023a/COMMANDER (ANGLE MODE)/STATE MACHINE SIGNALS/Generate Warning Messages for Console ==
  time (s) : Inport
  errors [8] : Inport  Port=2
  Boolean Value-Based Triggered Print : Subsystem  TreatAsAtomicUnit=on
  Matrix Concatenate : Concatenate  NumInputs=9  Mode=Multidimensional array  ConcatenateDimension=2
  String Constant : quarc_library/Strings/String Constant  string_value=Commander: Low Battery  evaluate_string=off  string_type=text  max_length=80  sample_time=inf  variable_size=off
      settings: AttributesFormatString="\"Commander: Low Battery\""  SourceProductName=QUARC Targets
  String Constant1 : quarc_library/Strings/String Constant  string_value=Commander: Sensor Failure  evaluate_string=off  string_type=text  max_length=80  sample_time=inf  variable_size=off
      settings: AttributesFormatString="\"Commander: Sensor Failure\""  SourceProductName=QUARC Targets
  String Constant2 : quarc_library/Strings/String Constant  string_value=Commander: Host Stream Issue / Problem with communication  evaluate_string=off  string_type=text  max_length=80  sample_time=inf  variable_size=off
      settings: AttributesFormatString="\"Commander: Host Stream Issue / Problem with communication\""  SourceProductName=QUARC Targets
  String Constant3 : quarc_library/Strings/String Constant  string_value=Commander: Joystick Issue  evaluate_string=off  string_type=text  max_length=80  sample_time=inf  variable_size=off
      settings: AttributesFormatString="\"Commander: Joystick Issue\""  SourceProductName=QUARC Targets
  String Constant4 : quarc_library/Strings/String Constant  string_value=Commander: Optitrack isn't tracking  evaluate_string=off  string_type=text  max_length=80  sample_time=inf  variable_size=off
      settings: AttributesFormatString="\"Commander: Optitrack isn't tracking\""  SourceProductName=QUARC Targets
  String Constant5 : quarc_library/Strings/String Constant  string_value=Commander: Flying low  evaluate_string=off  string_type=text  max_length=80  sample_time=inf  variable_size=off
      settings: AttributesFormatString="\"Commander: Flying low\""  SourceProductName=QUARC Targets
  String Constant6 : quarc_library/Strings/String Constant  string_value=Commander: Flying high  evaluate_string=off  string_type=text  max_length=80  sample_time=inf  variable_size=off
      settings: AttributesFormatString="\"Commander: Flying high\""  SourceProductName=QUARC Targets
  String Constant7 : quarc_library/Strings/String Constant  string_value=Commander: Emergency Stop Triggered  evaluate_string=off  string_type=text  max_length=80  sample_time=inf  variable_size=off
      settings: AttributesFormatString="\"Commander: Emergency Stop Triggered\""  SourceProductName=QUARC Targets
  String Constant8 : quarc_library/Strings/String Constant  string_value=Commander: Takeoff triggered before armed drone  evaluate_string=off  string_type=text  max_length=80  sample_time=inf  variable_size=off
      settings: AttributesFormatString="\"Commander: Takeoff triggered before armed drone\""  SourceProductName=QUARC Targets
  Terminator : Terminator
  wires:
  String Constant8/1 -> Matrix Concatenate/5
  String Constant4/1 -> Matrix Concatenate/6
  String Constant5/1 -> Matrix Concatenate/7
  String Constant6/1 -> Matrix Concatenate/8
  String Constant7/1 -> Matrix Concatenate/9
  Boolean Value-Based Triggered Print/1(Out1) -> Terminator/1
  String Constant3/1 -> Matrix Concatenate/4
  String Constant2/1 -> Matrix Concatenate/3
  String Constant1/1 -> Matrix Concatenate/2
  String Constant/1 -> Matrix Concatenate/1
  Matrix Concatenate/1 -> Boolean Value-Based Triggered Print/2(Message)
  errors [8]/1 -> Boolean Value-Based Triggered Print/1(Signal Enable)
  time (s)/1 -> Boolean Value-Based Triggered Print/3(time (s))

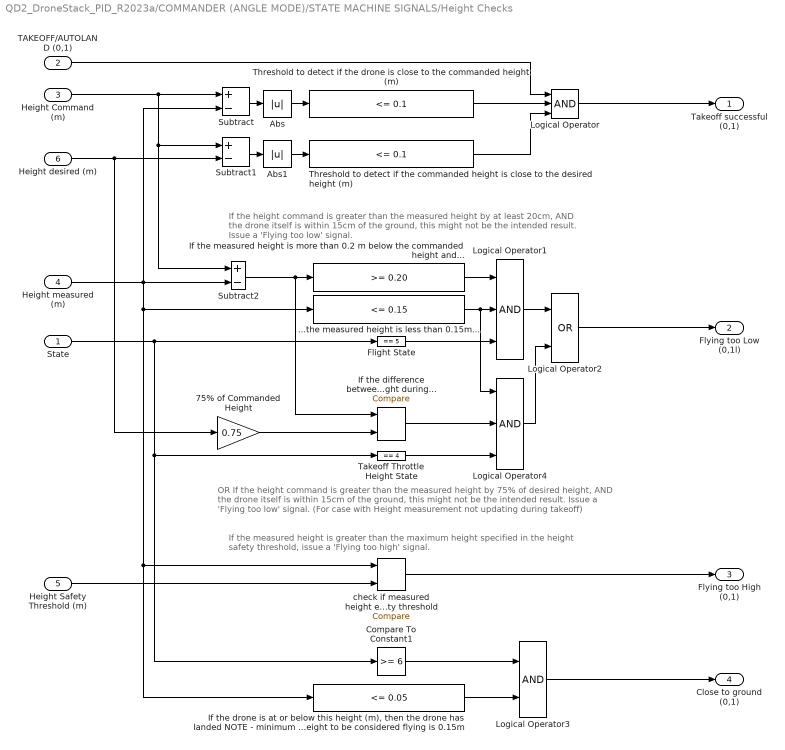
== system QD2_DroneStack_PID_R2023a/COMMANDER (ANGLE MODE)/STATE MACHINE SIGNALS/Height Checks ==
  note: OR If the height command is greater than the measured height by 75% of desired height, AND
      | the drone itself is within 15cm of the ground, this might not be the intended result. Issue a 'Flying too low' signal.
      | (For case with Height measurement not updating during takeoff)
  note: If the measured height is greater than the maximum height specified in the height safety threshold,
      | issue a 'Flying too high' signal.
  note: If the height command is greater than the measured height by at least 20cm, AND the drone itself is
      | within 15cm of the ground, this might not be the intended result. Issue a 'Flying too low' signal.
  State : Inport
  TAKEOFF/AUTOLAND (0,1) : Inport  Port=2
  Height Command (m) : Inport  Port=3
  Height measured (m) : Inport  Port=4
  Height Safety Threshold (m) : Inport  Port=5
  Height desired (m) : Inport  Port=6
  ...the measured height is less than 0.15m... : simulink/Logic and Bit Operations/Compare To Constant  relop=<=  const=0.15  OutDataTypeStr=boolean
  75% of Commanded Height : Gain  Gain=0.75
  Abs : Abs  SaturateOnIntegerOverflow=off
  Abs1 : Abs  SaturateOnIntegerOverflow=off
  Compare To Constant1 : simulink/Logic and Bit Operations/Compare To Constant  relop=>=  const=6  OutDataTypeStr=boolean
  Flight State : simulink/Logic and Bit Operations/Compare To Constant  relop===  const=5  OutDataTypeStr=boolean
  If the difference between the measured and commanded height is greater than 75% of the commanded height during... : quarc_library/Logic Operations/Compare  operator=>=  output_data_type=boolean
      settings: SourceProductName=QUARC Targets
  "If the drone is at or below this height (m), then the drone has landed NOTE - minimum height to be considered flying is 0.15m   " : simulink/Logic and Bit Operations/Compare To Constant  relop=<=  const=0.05  OutDataTypeStr=boolean
  If the measured height is more than 0.2 m below the commanded height and... : simulink/Logic and Bit Operations/Compare To Constant  relop=>=  const=0.20  OutDataTypeStr=boolean
  Logical Operator : Logic  Inputs=3  AllPortsSameDT=off  OutDataTypeStr=boolean
  Logical Operator1 : Logic  Inputs=3  AllPortsSameDT=off  OutDataTypeStr=boolean
  Logical Operator2 : Logic  Operator=OR  AllPortsSameDT=off  OutDataTypeStr=boolean
  Logical Operator3 : Logic  AllPortsSameDT=off  OutDataTypeStr=boolean
  Logical Operator4 : Logic  Inputs=3  AllPortsSameDT=off  OutDataTypeStr=boolean
  Subtract : Sum  Inputs=+-
  Subtract1 : Sum  Inputs=+-
  Subtract2 : Sum  Inputs=+-
  Takeoff Throttle Height State : simulink/Logic and Bit Operations/Compare To Constant  relop===  const=4  OutDataTypeStr=boolean
  Threshold to detect if the commanded height is close to the desired height (m) : simulink/Logic and Bit Operations/Compare To Constant  relop=<=  const=0.1  OutDataTypeStr=boolean
  Threshold to detect if the drone is close to the commanded height (m) : simulink/Logic and Bit Operations/Compare To Constant  relop=<=  const=0.1  OutDataTypeStr=boolean
  check if measured height exceeds maximum height safety threshold : quarc_library/Logic Operations/Compare  operator=>=  output_data_type=boolean
      settings: SourceProductName=QUARC Targets
  Takeoff successful (0,1) : Outport  VectorParamsAs1DForOutWhenUnconnected=off
  Flying too Low (0,1l) : Outport  Port=2  VectorParamsAs1DForOutWhenUnconnected=off
  Flying too High (0,1) : Outport  Port=3  VectorParamsAs1DForOutWhenUnconnected=off
  Close to ground (0,1) : Outport  Port=4  VectorParamsAs1DForOutWhenUnconnected=off
  wires:
  If the difference between the measured and commanded height is greater than 75% of the commanded height during.../1 -> Logical Operator4/2
  75% of Commanded Height/1 -> If the difference between the measured and commanded height is greater than 75% of the commanded height during.../2
  Takeoff Throttle Height State/1 -> Logical Operator4/3
  Subtract2/1 -> If the measured height is more than 0.2 m below the commanded height and.../1, If the difference between the measured and commanded height is greater than 75% of the commanded height during.../1
  Flight State/1 -> Logical Operator1/3
  Logical Operator4/1 -> Logical Operator2/2
  Height measured (m)/1 -> Subtract2/2, check if measured height exceeds maximum height safety threshold/1, "If the drone is at or below this height (m), then the drone has landed NOTE - minimum height to be considered flying is 0.15m   "/1, ...the measured height is less than 0.15m.../1, Subtract/2
  Compare To Constant1/1 -> Logical Operator3/1
  "If the drone is at or below this height (m), then the drone has landed NOTE - minimum height to be considered flying is 0.15m   "/1 -> Logical Operator3/2
  Logical Operator3/1 -> Close to ground (0,1)/1
  State/1 -> Compare To Constant1/1, Takeoff Throttle Height State/1, Flight State/1
  Height Safety Threshold (m)/1 -> check if measured height exceeds maximum height safety threshold/2
  check if measured height exceeds maximum height safety threshold/1 -> Flying too High (0,1)/1
  ...the measured height is less than 0.15m.../1 -> Logical Operator1/2, Logical Operator4/1
  Height Command (m)/1 -> Subtract/1, Subtract2/1, Subtract1/1
  Logical Operator1/1 -> Logical Operator2/1
  If the measured height is more than 0.2 m below the commanded height and.../1 -> Logical Operator1/1
  Subtract/1 -> Abs/1
  TAKEOFF/AUTOLAND (0,1)/1 -> Logical Operator/1
  Height desired (m)/1 -> Subtract1/2, 75% of Commanded Height/1
  Abs1/1 -> Threshold to detect if the commanded height is close to the desired height (m)/1
  Threshold to detect if the drone is close to the commanded height (m)/1 -> Logical Operator/2
  Abs/1 -> Threshold to detect if the drone is close to the commanded height (m)/1
  Threshold to detect if the commanded height is close to the desired height (m)/1 -> Logical Operator/3
  Subtract1/1 -> Abs1/1
  Logical Operator2/1 -> Flying too Low (0,1l)/1
  Logical Operator/1 -> Takeoff successful (0,1)/1

== system QD2_DroneStack_PID_R2023a/COMMANDER (ANGLE MODE)/STATE MACHINE SIGNALS/Latch E-Stop ==
  Input : Inport
  Trigger : TriggerPort  VariantControl=Variant
  Latched Output : Outport  InitialOutput=0  VectorParamsAs1DForOutWhenUnconnected=off
  wires:
  Input/1 -> Latched Output/1
